simulink model "gimbal_model_PID_180119"  (R2018b)
settings: Solver=FixedStepAuto  StartTime=0.0  StopTime=50  FixedStep=0.005  RelTol=1e-3
values from neighbouring files (symbols this model uses):
  DIM = data{4}    [gimbal_dynamics.m]
  DIS = data{5}    [gimbal_dynamics.m]
  F = 5e-5    (= 5e-05)    [BLDC_simulator.m]    (also in engine_parameters.m; engine_parameters_20191210.m = 1)
  I1 = data{1}    [gimbal_dynamics.m]    (also in macierze_inercji.m = sym('I1', [4 4]))
  I2 = data{2}    [gimbal_dynamics.m]    (also in macierze_inercji.m = sym('I2', [4 4]))
  I3 = data{3}    [gimbal_dynamics.m]    (also in macierze_inercji.m = sym('I3', [4 4]))
  J = 7.22e-6    (= 7.22e-06)    [BLDC_simulator.m]    (also in IMU.m = [cos(theta_2)*cos(theta_3) sin(theta_3) 0; engine_parameters.m; engine_parameters_20191210.m = 0.001)
  Kt = 8.44e-3    (= 0.00844)    [BLDC_simulator.m]    (also in engine_parameters.m)
  Kv = 8.44e-3    (= 0.00844)    [BLDC_simulator.m]    (also in engine_parameters.m)
  L = 0.42e-3    (= 0.00042)    [BLDC_simulator.m]    (also in engine_parameters.m; engine_parameters_20191210.m = 0.0005)
  M = [ud_ucz(3:p-1) ud_ucz(3:p-1).^2 ud_ucz(3:p-1).^3 ud_ucz(2:p-2) ud_ucz(2:p-2).^2 ud_ucz(2:p-2).^3 ud_ucz(1:p-3) ud_ucz(1:p-3).^2 ud_ucz(1:p-3).^3 yd_ucz(3:p-1) yd_ucz(3:p-1).^2 yd_ucz(3:p-1).^3 yd_ucz(2:p-2) yd_ucz(2:p-2).^2 yd_ucz(2:p-2).^3 yd_ucz(1:p-3) yd_ucz(1:p-3).^2 yd_ucz(1:p-3).^3]    [Identification_20191023.m]    (also in MI_beta.m = fillmissing(M,'spline'); gimbal_dynamics.m = data{6}; macierze_inercji.m = sym('M', [1 3]))
  R = 7.9    [BLDC_simulator.m]    (also in engine_parameters.m; engine_parameters_20191210.m = 0.5; inversekinematics.m = Rg*Rd*Rm)
libraries: simulink_extras x8, simulink x6
settings Model: Creator=Paweł Tymiński  LastModifiedBy=Paweł Tymiński
settings SolverCC: ZeroCrossAlgorithm=Adaptive
settings DebuggingCC: IgnoredZcDiagnostic=none
settings SFSimCC: SimUseLocalCustomCode=off
settings RTWCC: RTWUseLocalCustomCode=off
settings CodeAppCC: StateflowObjectComments=on
settings SimscapeCC: SimscapeNormalizeSystem=off

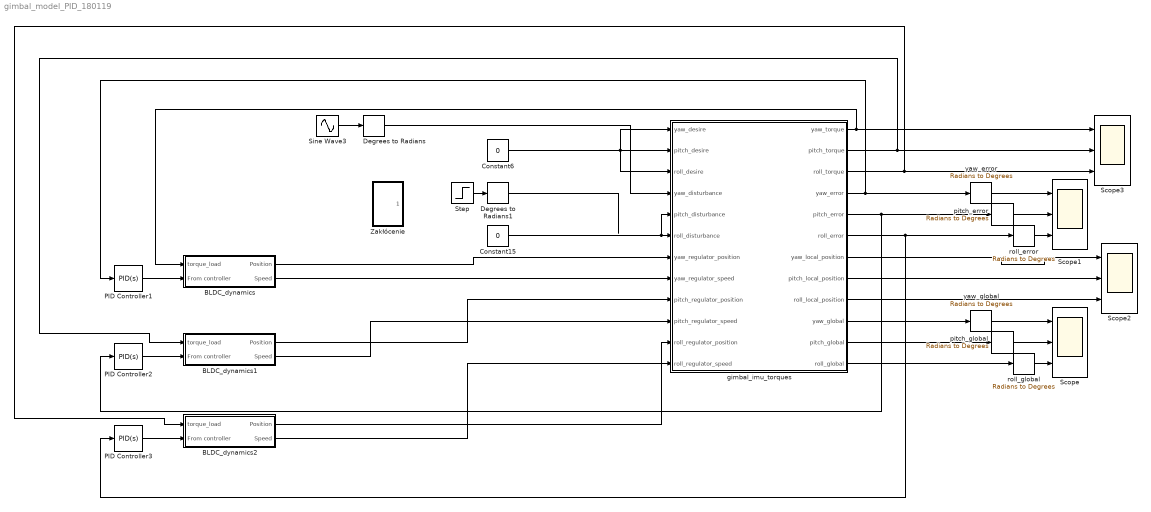
== system gimbal_model_PID_180119 ==
  BLDC_dynamics : Subsystem
  BLDC_dynamics1 : Subsystem
  BLDC_dynamics2 : Subsystem
  Constant15 : Constant  Value=0
  Constant6 : Constant  Value=0
  Degrees to Radians : simulink_extras/Transformations/Degrees to Radians
  Degrees to Radians1 : simulink_extras/Transformations/Degrees to Radians
  PID Controller1 : simulink/Continuous/PID Controller  Controller=PID  Form=Ideal  TimeDomain=Continuous-time  SampleTime=-1  IntegratorMethod=Forward Euler  FilterMethod=Forward Euler  ControllerParametersSource=internal  P=5.84311548545202  I=6.04781453430887  D=1.07517045237489  UseFilter=on  N=18169.6499905749  TunerSelectOption=Transfer Function Based (PID Tuner App)  InitialConditionSource=internal  InitialConditionForIntegrator=0  InitialConditionForFilter=0  DifferentiatorICPrevScaledInput=0  ExternalReset=none  TrackingMode=off  Kt=1  LimitOutput=off  UpperSaturationLimit=inf  LowerSaturationLimit=-inf  LinearizeAsGain=on  AntiWindupMode=none  Kb=1  POutMin=[]  POutMax=[]  IOutMin=[]  IOutMax=[]  DOutMin=[]  DOutMax=[]  NOutMin=[]  NOutMax=[]  SumOutMin=[]  SumOutMax=[]  SaturationOutMin=[]  SaturationOutMax=[]  PParamMin=[]  PParamMax=[]  IParamMin=[]  IParamMax=[]  DParamMin=[]  DParamMax=[]  NParamMin=[]  NParamMax=[]  KbParamMin=[]  KbParamMax=[]  KtParamMin=[]  KtParamMax=[]  KbOutMin=[]  KbOutMax=[]  KtOutMin=[]  KtOutMax=[]  IntegratorOutMin=[]  IntegratorOutMax=[]  FilterOutMin=[]  FilterOutMax=[]  SumI1OutMin=[]  SumI1OutMax=[]  SumI2OutMin=[]  SumI2OutMax=[]  SumI3OutMin=[]  SumI3OutMax=[]  SumI4OutMin=[]  SumI4OutMax=[]  SumDOutMin=[]  SumDOutMax=[]  DifferentiatorOutMin=[]  DifferentiatorOutMax=[]  FilterDiffOutCoefMin=[]  FilterDiffOutCoefMax=[]  ReciprocalOutMin=[]  ReciprocalOutMax=[]  SumDenOutMin=[]  SumDenOutMax=[]  SumNumOutMin=[]  SumNumOutMax=[]  DivideOutMin=[]  DivideOutMax=[]  IntegratorContinuousStateAttributes=''  IntegratorStateMustResolveToSignalObject=off  IntegratorRTWStateStorageClass=Auto  FilterContinuousStateAttributes=''  FilterStateMustResolveToSignalObject=off  FilterRTWStateStorageClass=Auto  ParallelPVariant=Passthrough  IdealPVariant=InternalParameters  IVariant=InternalParameters  DVariant=InternalParameters  IntegratorVariant=Continuous  SatVariant=Disabled  AWVariant=Passthrough  PCopyVariant=Disabled  TRVariant=Disabled  FdbkBlocksVariant=Forward  IdealPFdbkVariant=Disabled  SatFdbkVariant=Disabled  DerivativeFilterVariant=ContFilter  NVariant=InternalParameters  NCopyVariant=Disabled  FilterICVariant=InternalICsFilter  IntegratorICVariant=InternalICs  ExternalResetVariant=Disabled  TRSumVariant=Passthrough  SumFdbkVariant=Disabled  SumVariant=Sum_PID
  PID Controller2 : simulink/Continuous/PID Controller  Controller=PID  Form=Ideal  TimeDomain=Continuous-time  SampleTime=-1  IntegratorMethod=Forward Euler  FilterMethod=Forward Euler  ControllerParametersSource=internal  P=4510.14665537274  I=28.9272498505744  D=0.00768093030791191  UseFilter=on  N=566665.638352997  TunerSelectOption=Transfer Function Based (PID Tuner App)  InitialConditionSource=internal  InitialConditionForIntegrator=0  InitialConditionForFilter=0  DifferentiatorICPrevScaledInput=0  ExternalReset=none  TrackingMode=off  Kt=1  LimitOutput=off  UpperSaturationLimit=inf  LowerSaturationLimit=-inf  LinearizeAsGain=on  AntiWindupMode=none  Kb=1  POutMin=[]  POutMax=[]  IOutMin=[]  IOutMax=[]  DOutMin=[]  DOutMax=[]  NOutMin=[]  NOutMax=[]  SumOutMin=[]  SumOutMax=[]  SaturationOutMin=[]  SaturationOutMax=[]  PParamMin=[]  PParamMax=[]  IParamMin=[]  IParamMax=[]  DParamMin=[]  DParamMax=[]  NParamMin=[]  NParamMax=[]  KbParamMin=[]  KbParamMax=[]  KtParamMin=[]  KtParamMax=[]  KbOutMin=[]  KbOutMax=[]  KtOutMin=[]  KtOutMax=[]  IntegratorOutMin=[]  IntegratorOutMax=[]  FilterOutMin=[]  FilterOutMax=[]  SumI1OutMin=[]  SumI1OutMax=[]  SumI2OutMin=[]  SumI2OutMax=[]  SumI3OutMin=[]  SumI3OutMax=[]  SumI4OutMin=[]  SumI4OutMax=[]  SumDOutMin=[]  SumDOutMax=[]  DifferentiatorOutMin=[]  DifferentiatorOutMax=[]  FilterDiffOutCoefMin=[]  FilterDiffOutCoefMax=[]  ReciprocalOutMin=[]  ReciprocalOutMax=[]  SumDenOutMin=[]  SumDenOutMax=[]  SumNumOutMin=[]  SumNumOutMax=[]  DivideOutMin=[]  DivideOutMax=[]  IntegratorContinuousStateAttributes=''  IntegratorStateMustResolveToSignalObject=off  IntegratorRTWStateStorageClass=Auto  FilterContinuousStateAttributes=''  FilterStateMustResolveToSignalObject=off  FilterRTWStateStorageClass=Auto  ParallelPVariant=Passthrough  IdealPVariant=InternalParameters  IVariant=InternalParameters  DVariant=InternalParameters  IntegratorVariant=Continuous  SatVariant=Disabled  AWVariant=Passthrough  PCopyVariant=Disabled  TRVariant=Disabled  FdbkBlocksVariant=Forward  IdealPFdbkVariant=Disabled  SatFdbkVariant=Disabled  DerivativeFilterVariant=ContFilter  NVariant=InternalParameters  NCopyVariant=Disabled  FilterICVariant=InternalICsFilter  IntegratorICVariant=InternalICs  ExternalResetVariant=Disabled  TRSumVariant=Passthrough  SumFdbkVariant=Disabled  SumVariant=Sum_PID
  PID Controller3 : simulink/Continuous/PID Controller  Controller=PID  Form=Ideal  TimeDomain=Continuous-time  SampleTime=-1  IntegratorMethod=Forward Euler  FilterMethod=Forward Euler  ControllerParametersSource=internal  P=796.461585317197  I=12.3206342172023  D=0.0180338273326542  UseFilter=on  N=241353.052560096  TunerSelectOption=Transfer Function Based (PID Tuner App)  InitialConditionSource=internal  InitialConditionForIntegrator=0  InitialConditionForFilter=0  DifferentiatorICPrevScaledInput=0  ExternalReset=none  TrackingMode=off  Kt=1  LimitOutput=off  UpperSaturationLimit=inf  LowerSaturationLimit=-inf  LinearizeAsGain=on  AntiWindupMode=none  Kb=1  POutMin=[]  POutMax=[]  IOutMin=[]  IOutMax=[]  DOutMin=[]  DOutMax=[]  NOutMin=[]  NOutMax=[]  SumOutMin=[]  SumOutMax=[]  SaturationOutMin=[]  SaturationOutMax=[]  PParamMin=[]  PParamMax=[]  IParamMin=[]  IParamMax=[]  DParamMin=[]  DParamMax=[]  NParamMin=[]  NParamMax=[]  KbParamMin=[]  KbParamMax=[]  KtParamMin=[]  KtParamMax=[]  KbOutMin=[]  KbOutMax=[]  KtOutMin=[]  KtOutMax=[]  IntegratorOutMin=[]  IntegratorOutMax=[]  FilterOutMin=[]  FilterOutMax=[]  SumI1OutMin=[]  SumI1OutMax=[]  SumI2OutMin=[]  SumI2OutMax=[]  SumI3OutMin=[]  SumI3OutMax=[]  SumI4OutMin=[]  SumI4OutMax=[]  SumDOutMin=[]  SumDOutMax=[]  DifferentiatorOutMin=[]  DifferentiatorOutMax=[]  FilterDiffOutCoefMin=[]  FilterDiffOutCoefMax=[]  ReciprocalOutMin=[]  ReciprocalOutMax=[]  SumDenOutMin=[]  SumDenOutMax=[]  SumNumOutMin=[]  SumNumOutMax=[]  DivideOutMin=[]  DivideOutMax=[]  IntegratorContinuousStateAttributes=''  IntegratorStateMustResolveToSignalObject=off  IntegratorRTWStateStorageClass=Auto  FilterContinuousStateAttributes=''  FilterStateMustResolveToSignalObject=off  FilterRTWStateStorageClass=Auto  ParallelPVariant=Passthrough  IdealPVariant=InternalParameters  IVariant=InternalParameters  DVariant=InternalParameters  IntegratorVariant=Continuous  SatVariant=Disabled  AWVariant=Passthrough  PCopyVariant=Disabled  TRVariant=Disabled  FdbkBlocksVariant=Forward  IdealPFdbkVariant=Disabled  SatFdbkVariant=Disabled  DerivativeFilterVariant=ContFilter  NVariant=InternalParameters  NCopyVariant=Disabled  FilterICVariant=InternalICsFilter  IntegratorICVariant=InternalICs  ExternalResetVariant=Disabled  TRSumVariant=Passthrough  SumFdbkVariant=Disabled  SumVariant=Sum_PID
  Scope{,1..3} (4 alike) : Scope  NumInputPorts=3
  Sine Wave3 : Sin  Amplitude=15  Frequency=0.25*pi  SampleTime=0
  Step : Step  Time=2  After=10  SampleTime=0
  Zakłócenie : Subsystem
  gimbal_imu_torques : Subsystem
  pitch_error : simulink_extras/Transformations/Radians to Degrees
  pitch_global : simulink_extras/Transformations/Radians to Degrees
  roll_error : simulink_extras/Transformations/Radians to Degrees
  roll_global : simulink_extras/Transformations/Radians to Degrees
  yaw_error : simulink_extras/Transformations/Radians to Degrees
  yaw_global : simulink_extras/Transformations/Radians to Degrees
  wires:
  Constant6/1 -> gimbal_imu_torques/3(roll_desire), gimbal_imu_torques/2(pitch_desire), gimbal_imu_torques/1(yaw_desire)
  gimbal_imu_torques/1(yaw_torque) -> Scope3/1, BLDC_dynamics/1(torque_load)
  gimbal_imu_torques/4(yaw_error) -> yaw_error/1, PID Controller1/1
  BLDC_dynamics/1(Position) -> gimbal_imu_torques/7(yaw_regulator_position)
  BLDC_dynamics/2(Speed) -> gimbal_imu_torques/8(yaw_regulator_speed)
  PID Controller1/1 -> BLDC_dynamics/2(From controller)
  PID Controller2/1 -> BLDC_dynamics1/2(From controller)
  PID Controller3/1 -> BLDC_dynamics2/2(From controller)
  gimbal_imu_torques/2(pitch_torque) -> Scope3/2, BLDC_dynamics1/1(torque_load)
  gimbal_imu_torques/3(roll_torque) -> Scope3/3, BLDC_dynamics2/1(torque_load)
  gimbal_imu_torques/6(roll_error) -> roll_error/1, PID Controller3/1
  gimbal_imu_torques/11(pitch_global) -> pitch_global/1
  gimbal_imu_torques/10(yaw_global) -> yaw_global/1
  gimbal_imu_torques/12(roll_global) -> roll_global/1
  Sine Wave3/1 -> Degrees to Radians/1
  gimbal_imu_torques/5(pitch_error) -> PID Controller2/1, pitch_error/1
  yaw_error/1 -> Scope1/1
  roll_global/1 -> Scope/3
  pitch_global/1 -> Scope/2
  yaw_global/1 -> Scope/1
  roll_error/1 -> Scope1/3
  pitch_error/1 -> Scope1/2
  gimbal_imu_torques/8(pitch_local_position) -> Scope2/2
  gimbal_imu_torques/7(yaw_local_position) -> Scope2/1
  gimbal_imu_torques/9(roll_local_position) -> Scope2/3
  Constant15/1 -> gimbal_imu_torques/5(pitch_disturbance), gimbal_imu_torques/6(roll_disturbance)
  BLDC_dynamics2/1(Position) -> gimbal_imu_torques/11(roll_regulator_position)
  BLDC_dynamics2/2(Speed) -> gimbal_imu_torques/12(roll_regulator_speed)
  BLDC_dynamics1/1(Position) -> gimbal_imu_torques/9(pitch_regulator_position)
  BLDC_dynamics1/2(Speed) -> gimbal_imu_torques/10(pitch_regulator_speed)
  Step/1 -> Degrees to Radians1/1
  Degrees to Radians1/1 -> ?
  Degrees to Radians/1 -> gimbal_imu_torques/4(yaw_disturbance)

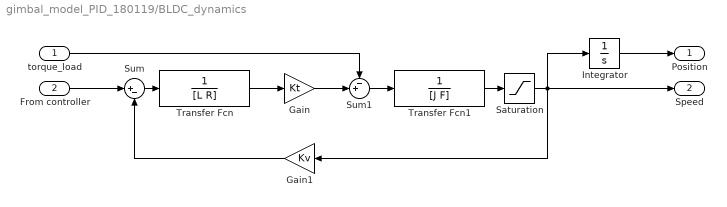
== system gimbal_model_PID_180119/BLDC_dynamics ==
  torque_load : Inport
  From controller : Inport  Port=2
  Gain : Gain  Gain=Kt
  Gain1 : Gain  Gain=Kv
  Integrator : Integrator
  Saturation : Saturate  UpperLimit=2*pi  LowerLimit=-2*pi
  Sum : Sum  Inputs=|+-
  Sum1 : Sum  Inputs=-+|
  Transfer Fcn : TransferFcn  Denominator=[L R]
  Transfer Fcn1 : TransferFcn  Denominator=[J F]
  Position : Outport
  Speed : Outport  Port=2
  wires:
  Gain/1 -> Sum1/2
  Transfer Fcn1/1 -> Saturation/1
  Transfer Fcn/1 -> Gain/1
  Sum/1 -> Transfer Fcn/1
  From controller/1 -> Sum/1
  torque_load/1 -> Sum1/1
  Gain1/1 -> Sum/2
  Sum1/1 -> Transfer Fcn1/1
  Integrator/1 -> Position/1
  Saturation/1 -> Integrator/1, Gain1/1, Speed/1

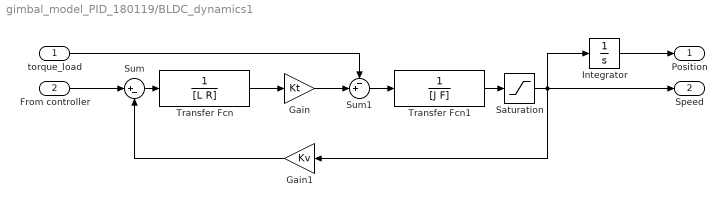
== system gimbal_model_PID_180119/BLDC_dynamics1 ==
  torque_load : Inport
  From controller : Inport  Port=2
  Gain : Gain  Gain=Kt
  Gain1 : Gain  Gain=Kv
  Integrator : Integrator
  Saturation : Saturate  UpperLimit=2*pi  LowerLimit=-2*pi
  Sum : Sum  Inputs=|+-
  Sum1 : Sum  Inputs=-+|
  Transfer Fcn : TransferFcn  Denominator=[L R]
  Transfer Fcn1 : TransferFcn  Denominator=[J F]
  Position : Outport
  Speed : Outport  Port=2
  wires:
  Gain/1 -> Sum1/2
  Transfer Fcn1/1 -> Saturation/1
  Transfer Fcn/1 -> Gain/1
  Sum/1 -> Transfer Fcn/1
  From controller/1 -> Sum/1
  torque_load/1 -> Sum1/1
  Gain1/1 -> Sum/2
  Sum1/1 -> Transfer Fcn1/1
  Integrator/1 -> Position/1
  Saturation/1 -> Integrator/1, Gain1/1, Speed/1

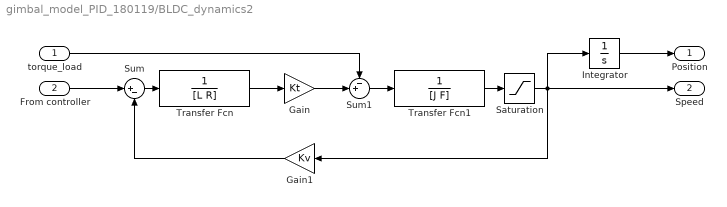
== system gimbal_model_PID_180119/BLDC_dynamics2 ==
  torque_load : Inport
  From controller : Inport  Port=2
  Gain : Gain  Gain=Kt
  Gain1 : Gain  Gain=Kv
  Integrator : Integrator
  Saturation : Saturate  UpperLimit=2*pi  LowerLimit=-2*pi
  Sum : Sum  Inputs=|+-
  Sum1 : Sum  Inputs=-+|
  Transfer Fcn : TransferFcn  Denominator=[L R]
  Transfer Fcn1 : TransferFcn  Denominator=[J F]
  Position : Outport
  Speed : Outport  Port=2
  wires:
  Gain/1 -> Sum1/2
  Transfer Fcn1/1 -> Saturation/1
  Transfer Fcn/1 -> Gain/1
  Sum/1 -> Transfer Fcn/1
  From controller/1 -> Sum/1
  torque_load/1 -> Sum1/1
  Gain1/1 -> Sum/2
  Sum1/1 -> Transfer Fcn1/1
  Integrator/1 -> Position/1
  Saturation/1 -> Integrator/1, Gain1/1, Speed/1

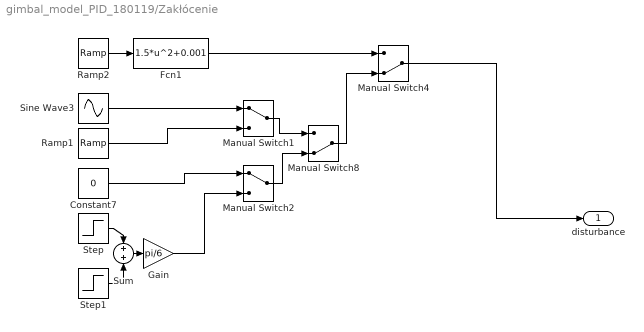
== system gimbal_model_PID_180119/Zakłócenie ==
  Constant7 : Constant  Value=0
  Fcn1 : Fcn  Expr=1.5*u^2+0.001
  Gain : Gain  Gain=pi/6
  Manual Switch1 : ManualSwitch
  Manual Switch2 : ManualSwitch
  Manual Switch4 : ManualSwitch  CurrentSetting=0
  Manual Switch8 : ManualSwitch  CurrentSetting=0
  Ramp1 : simulink/Sources/Ramp  slope=pi/16  start=0  InitialOutput=0
  Ramp2 : simulink/Sources/Ramp  slope=pi/8  start=0  InitialOutput=0
  Sine Wave3 : Sin  Amplitude=pi/18  SampleTime=0
  Step : Step  SampleTime=0
  Step1 : Step  Time=2  After=-1  SampleTime=0
  Sum : Sum
  disturbance : Outport
  wires:
  Sum/1 -> Gain/1
  Step1/1 -> Sum/2
  Manual Switch2/1 -> Manual Switch8/2
  Manual Switch1/1 -> Manual Switch8/1
  Constant7/1 -> Manual Switch2/1
  Step/1 -> Sum/1
  Manual Switch8/1 -> Manual Switch4/2
  Sine Wave3/1 -> Manual Switch1/1
  Gain/1 -> Manual Switch2/2
  Fcn1/1 -> Manual Switch4/1
  Ramp1/1 -> Manual Switch1/2
  Manual Switch4/1 -> disturbance/1
  Ramp2/1 -> Fcn1/1

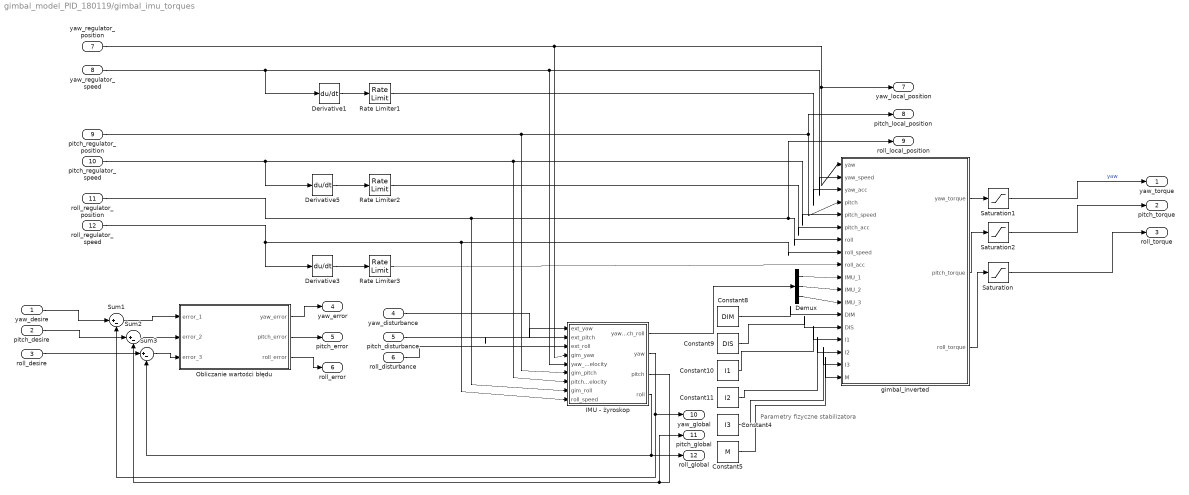
== system gimbal_model_PID_180119/gimbal_imu_torques ==
  note: Parametry fizyczne stabilizatora
  yaw_desire : Inport
  pitch_desire : Inport  Port=2
  roll_desire : Inport  Port=3
  yaw_disturbance : Inport  Port=4
  pitch_disturbance : Inport  Port=5
  roll_disturbance : Inport  Port=6
  yaw_regulator_position : Inport  Port=7
  yaw_regulator_speed : Inport  Port=8
  pitch_regulator_position : Inport  Port=9
  pitch_regulator_speed : Inport  Port=10
  roll_regulator_position : Inport  Port=11
  roll_regulator_speed : Inport  Port=12
  Constant10 : Constant  Value=I1
  Constant11 : Constant  Value=I2
  Constant4 : Constant  Value=I3
  Constant5 : Constant  Value=M
  Constant8 : Constant  Value=DIM
  Constant9 : Constant  Value=DIS
  Demux : Demux  Outputs=3
  Derivative1 : Derivative
  Derivative3 : Derivative
  Derivative5 : Derivative
  IMU - żyroskop : Subsystem
  Obliczanie wartości błędu : MATLAB Function  TreatAsAtomicUnit=on
  Rate Limiter1 : RateLimiter  RisingSlewLimit=25  FallingSlewLimit=-25  SampleTimeMode=inherited
  Rate Limiter2 : RateLimiter  RisingSlewLimit=25  FallingSlewLimit=-25  SampleTimeMode=inherited
  Rate Limiter3 : RateLimiter  RisingSlewLimit=25  FallingSlewLimit=-25  SampleTimeMode=inherited
  Saturation : Saturate  UpperLimit=10  LowerLimit=-10
  Saturation1 : Saturate  UpperLimit=10  LowerLimit=-10
  Saturation2 : Saturate  UpperLimit=10  LowerLimit=-10
  Sum1 : Sum  Inputs=|+-
  Sum2 : Sum  Inputs=|+-
  Sum3 : Sum  Inputs=|+-
  gimbal_inverted : MATLAB Function  TreatAsAtomicUnit=on
  yaw_torque : Outport
  pitch_torque : Outport  Port=2
  roll_torque : Outport  Port=3
  yaw_error : Outport  Port=4
  pitch_error : Outport  Port=5
  roll_error : Outport  Port=6
  yaw_local_position : Outport  Port=7
  pitch_local_position : Outport  Port=8
  roll_local_position : Outport  Port=9
  yaw_global : Outport  Port=10
  pitch_global : Outport  Port=11
  roll_global : Outport  Port=12
  wires:
  Demux/1 -> gimbal_inverted/10(IMU_1)
  roll_regulator_position/1 -> IMU - żyroskop/8("gim_roll "), gimbal_inverted/7(roll), roll_local_position/1
  Sum3/1 -> Obliczanie wartości błędu/3(error_3)
  pitch_regulator_position/1 -> IMU - żyroskop/6(gim_pitch), pitch_local_position/1, gimbal_inverted/4(pitch)
  gimbal_inverted/2(pitch_torque) -> Saturation2/1
  yaw_regulator_speed/1 -> Derivative1/1, IMU - żyroskop/5(yaw_velocity), gimbal_inverted/2(yaw_speed)
  Demux/2 -> gimbal_inverted/11(IMU_2)
  Rate Limiter1/1 -> gimbal_inverted/3(yaw_acc)
  IMU - żyroskop/1(yaw_pitch_roll) -> Demux/1
  Demux/3 -> gimbal_inverted/12(IMU_3)
  Rate Limiter3/1 -> gimbal_inverted/9(roll_acc)
  roll_regulator_speed/1 -> Derivative3/1, IMU - żyroskop/9(roll_speed), gimbal_inverted/8(roll_speed)
  pitch_regulator_speed/1 -> gimbal_inverted/5(pitch_speed), IMU - żyroskop/7(pitch_velocity), Derivative5/1
  Derivative5/1 -> Rate Limiter2/1
  Constant8/1 -> gimbal_inverted/13(DIM)
  Constant4/1 -> gimbal_inverted/17(I3)
  IMU - żyroskop/3(pitch) -> Sum2/2, pitch_global/1
  gimbal_inverted/3(roll_torque) -> Saturation/1
  Constant11/1 -> gimbal_inverted/16(I2)
  Sum2/1 -> Obliczanie wartości błędu/2(error_2)
  Derivative3/1 -> Rate Limiter3/1
  Sum1/1 -> Obliczanie wartości błędu/1(error_1)
  Derivative1/1 -> Rate Limiter1/1
  Constant5/1 -> gimbal_inverted/18(M)
  gimbal_inverted/1(yaw_torque) -> Saturation1/1
  Rate Limiter2/1 -> gimbal_inverted/6(pitch_acc)
  Constant10/1 -> gimbal_inverted/15(I1)
  pitch_disturbance/1 -> IMU - żyroskop/2(ext_pitch)
  IMU - żyroskop/4(roll) -> Sum3/2, roll_global/1
  IMU - żyroskop/2(yaw) -> Sum1/2, yaw_global/1
  Obliczanie wartości błędu/2(pitch_error) -> pitch_error/1
  roll_disturbance/1 -> IMU - żyroskop/3(ext_roll)
  Constant9/1 -> gimbal_inverted/14(DIS)
  yaw_disturbance/1 -> IMU - żyroskop/1(ext_yaw)
  Obliczanie wartości błędu/3(roll_error) -> roll_error/1
  Saturation/1 -> roll_torque/1
  Obliczanie wartości błędu/1(yaw_error) -> yaw_error/1
  Saturation2/1 -> pitch_torque/1
  Saturation1/1 -> yaw_torque/1  "yaw"
  yaw_desire/1 -> Sum1/1
  pitch_desire/1 -> Sum2/1
  roll_desire/1 -> Sum3/1
  yaw_regulator_position/1 -> yaw_local_position/1, gimbal_inverted/1(yaw), IMU - żyroskop/4(gim_yaw)

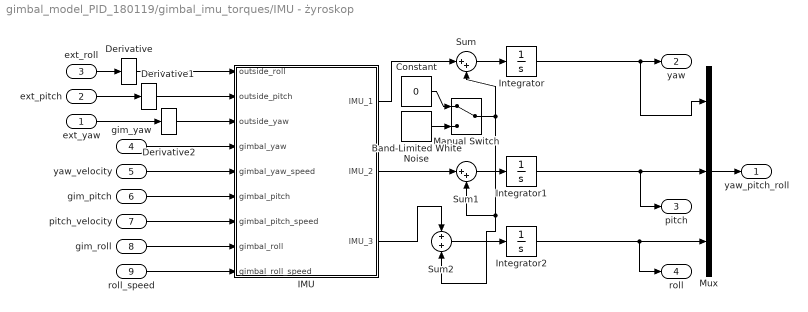
== system gimbal_model_PID_180119/gimbal_imu_torques/IMU - żyroskop ==
  ext_yaw : Inport
  ext_pitch : Inport  Port=2
  ext_roll : Inport  Port=3
  gim_yaw : Inport  Port=4
  yaw_velocity : Inport  Port=5
  gim_pitch : Inport  Port=6
  pitch_velocity : Inport  Port=7
  "gim_roll " : Inport  Port=8
  roll_speed : Inport  Port=9
  Band-Limited White Noise : simulink/Sources/Band-Limited White Noise  Cov=[0.1]  Ts=0.1  seed=[23341]
  Constant : Constant  Value=0
  Derivative : Derivative
  Derivative1 : Derivative
  Derivative2 : Derivative
  IMU : MATLAB Function  TreatAsAtomicUnit=on
  Integrator : Integrator
  Integrator1 : Integrator
  Integrator2 : Integrator
  Manual Switch : ManualSwitch
  Mux : Mux  Inputs=3
  Sum : Sum  Inputs=|++
  Sum1 : Sum  Inputs=|++
  Sum2 : Sum
  yaw_pitch_roll : Outport
  yaw : Outport  Port=2
  pitch : Outport  Port=3
  roll : Outport  Port=4
  wires:
  roll_speed/1 -> IMU/9(gimbal_roll_speed)
  gim_pitch/1 -> IMU/6(gimbal_pitch)
  Mux/1 -> yaw_pitch_roll/1
  yaw_velocity/1 -> IMU/5(gimbal_yaw_speed)
  IMU/1(IMU_1) -> Sum/1
  pitch_velocity/1 -> IMU/7(gimbal_pitch_speed)
  ext_pitch/1 -> Derivative1/1
  ext_roll/1 -> Derivative/1
  ext_yaw/1 -> Derivative2/1
  "gim_roll "/1 -> IMU/8(gimbal_roll)
  gim_yaw/1 -> IMU/4(gimbal_yaw)
  IMU/3(IMU_3) -> Sum2/1
  IMU/2(IMU_2) -> Sum1/1
  Manual Switch/1 -> Sum2/2, Sum1/2, Sum/2
  Sum2/1 -> Integrator2/1
  Sum1/1 -> Integrator1/1
  Sum/1 -> Integrator/1
  Band-Limited White Noise/1 -> Manual Switch/2
  Constant/1 -> Manual Switch/1
  Derivative/1 -> IMU/1(outside_roll)
  Derivative1/1 -> IMU/2(outside_pitch)
  Derivative2/1 -> IMU/3(outside_yaw)
  Integrator/1 -> Mux/1, yaw/1
  Integrator2/1 -> roll/1, Mux/3
  Integrator1/1 -> pitch/1, Mux/2

== matlab function gimbal_model_PID_180119/gimbal_imu_torques/IMU - żyroskop/IMU ==
  data: outside_roll input; IMU_1 output; outside_pitch input; outside_yaw input; gimbal_yaw input; gimbal_yaw_speed input; gimbal_pitch input; gimbal_pitch_speed input; gimbal_roll input; gimbal_roll_speed input; IMU_2 output; IMU_3 output

function [IMU_1, IMU_2, IMU_3] = IMU(outside_roll,outside_pitch,outside_yaw,gimbal_yaw ,gimbal_yaw_speed, gimbal_pitch ,gimbal_pitch_speed , gimbal_roll , gimbal_roll_speed  )
% kąty gimbala
theta_1 = gimbal_yaw ;
theta_2 = gimbal_pitch ;
theta_3 = gimbal_roll ;

J_0 =[1 0 0;
    0 cos(theta_1) -sin(theta_1);
   -sin(theta_2) cos(theta_2)*sin(theta_1) cos(theta_1)*cos(theta_2)];
Phi_0 = [outside_yaw; outside_pitch; outside_roll];

Omega_phi = J_0*Phi_0;

Omega = [gimbal_yaw_speed; gimbal_pitch_speed; gimbal_roll_speed];

J = [cos(theta_2)*cos(theta_3) sin(theta_3) 0;
    cos(theta_2)*sin(theta_3) cos(theta_3) 0;
    -sin(theta_2) 0 1];
A=J*(Omega_phi + Omega);

IMU_1 = A(1); %yaw
IMU_2 = A(2); %pitch
IMU_3 = A(3); %roll

end

== matlab function gimbal_model_PID_180119/gimbal_imu_torques/Obliczanie wartości błędu ==
  data: error_1 input; error_2 input; error_3 input; yaw_error output; pitch_error output; roll_error output
function [yaw_error, pitch_error, roll_error] = fcn(error_1,error_2,error_3)
E=[cos(error_1)*cos(error_3)-sin(error_1)*sin(error_2)*sin(error_3) -cos(error_2)*sin(error_1) cos(error_1)*sin(error_1)+cos(error_3)*sin(error_1)*sin(error_2);
cos(error_3)*sin(error_1)+cos(error_1)*sin(error_2)*sin(error_2) cos(error_1)*cos(error_2) sin(error_1)*sin(error_3)-cos(error_1)*cos(error_3)*sin(error_2);
-cos(error_2)*sin(error_3) sin(error_2) cos(error_2)*cos(error_3)];



r12 = E(1,2);
r22 = E(2,2);
r31 = E(3,1);
r32 = E(3,2);
r33 = E(3,3);
yaw_D=atan2(-r12,r22);
pitch_D=asin(r32);
roll_D=atan2(-r31,r33);
% yaw_error=yaw_D-yaw_L;
% pitch_error=pitch_D-pitch_L;
% roll_error=roll_D-roll_L;

yaw_error=yaw_D;
pitch_error=pitch_D;
roll_error=roll_D;
end

== matlab function gimbal_model_PID_180119/gimbal_imu_torques/gimbal_inverted ==
  data: yaw input; yaw_speed input; yaw_acc input; pitch input; pitch_speed input; pitch_acc input; roll input; yaw_torque output; roll_speed input; roll_acc input; IMU_1 input; IMU_2 input; IMU_3 input; DIM input; DIS input; I1 input; I2 input; I3 input; M input; pitch_torque output; roll_torque output
function [yaw_torque, pitch_torque, roll_torque]  = gimbal_dynamics(yaw,yaw_speed,yaw_acc,pitch,pitch_speed,pitch_acc,roll,roll_speed, roll_acc,IMU_1,IMU_2,IMU_3,DIM,DIS,I1,I2,I3,M)

%stała grawitacji
g = 9.81;


%-------------ZMIENNE--------------
% odczyty z IMU
alpha_1 = IMU_1;
alpha_2 = IMU_2;
alpha_3 = IMU_3;
IMU = [alpha_1; alpha_2; alpha_3];
%predkosci katowe osiagane przez gimbal
 om_1 = yaw_speed ;
 om_2 = pitch_speed ;
 om_3 = roll_speed ;
Omega = [om_1; om_2; om_3];
%kąty osiagane aktualnie przez gimbal
 theta_1 = yaw ;
 theta_2 = pitch ;
 theta_3 = roll ;
 THETA = [theta_1; theta_2; theta_3];
% przyśpieszenia kątowe w osiach gimbala
 ACC = [yaw_acc;pitch_acc;roll_acc];

%---------------FUNKCJE---------------------

H = calculate_H_matrix(THETA,Omega,I1,I2,I3,DIM);
D = calculate_D_matrix(THETA,I1,I2,I3,DIM);
G = calculate_G_matrix(IMU,THETA,DIM,g,M,DIS);
Q = D*ACC+H+G;
yaw_torque = Q(1);
pitch_torque = Q(2);
roll_torque = Q(3);

end
